simulink model "Lab8_model_12a"  (R2012a)
settings: Solver=ode45  StartTime=0.0  StopTime=20  RelTol=1e-3
values from neighbouring files (symbols this model uses):
  A = [0 4 2;0 0 2;6 2 3]    [Lab8.m]
  B = [3;0;0]    [Lab8.m]
  C = [4 1 2]    [Lab8.m]
  D = 0    [Lab8.m]
  K = 0.02    [Controle_Lab4.m]    (also in Lab8.m = place(A,B,[-10 -12 -2]); Tarefa1.m)
  K1 = 9    [Lab8.m]
  K2 = 11    [Lab8.m]
  K3 = 14.5    [Lab8.m]
settings Model: Creator=11104980  LastModifiedBy=Jessica
settings DataIOCC: LimitDataPoints=on  SaveFormat=Array  ReturnWorkspaceOutputs=off
settings OptimizationCC: ExpressionDepthLimit=2147483647  LifeSpan=inf  SimCompilerOptimization=Off
settings DebuggingCC: UnderspecifiedInitializationDetection=Classic  MergeDetectMultiDrivingBlocksExec=none  FcnCallInpInsideContextMsg=Enable All  StateNameClashWarn=warning  SFUnexpectedBacktrackingDiag=warning  SFNoUnconditionalDefaultTransitionDiag=warning
settings HardwareCC: ProdBitPerPointer=32  ProdLargestAtomicFloat=None  ProdIntDivRoundTo=Undefined  ProdEndianess=Unspecified  ProdWordSize=32  ProdHWDeviceType=32-bit Generic
settings ModelReferenceCC: PropagateSignalLabelsOutOfModel=off
settings SFSimCC: SimUseLocalCustomCode=off
settings RTWCC: RTWUseLocalCustomCode=off  RTWCompilerOptimization=Off
settings GRTTargetCC: CodeReplacementLibrary=C89/C90 (ANSI)  GeneratePreprocessorConditionals=Disable all  CPPClassGenCompliant=off

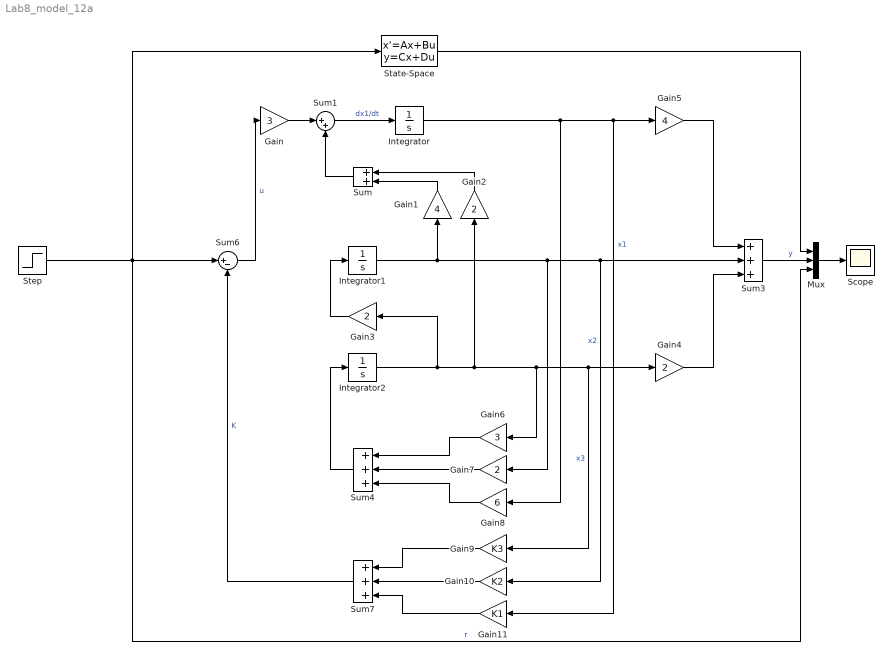
== system Lab8_model_12a ==
  Gain : Gain  Gain=3
  Gain1 : Gain  Gain=4
  Gain10 : Gain  Gain=K2
  Gain11 : Gain  Gain=K1
  Gain{2..4,7} (4 alike) : Gain  Gain=2
  Gain5 : Gain  Gain=4
  Gain6 : Gain  Gain=3
  Gain8 : Gain  Gain=6
  Gain9 : Gain  Gain=K3
  Integrator : Integrator
  Integrator1 : Integrator
  Integrator2 : Integrator
  Mux : Mux  Inputs=3
  Scope : Scope
      settings: SaveName=y
  State-Space : StateSpace  A=(A-B*K)  B=B  C=C  D=D  X0=0
  Step : Step  SampleTime=0
  Sum : Sum
  Sum1 : Sum  Inputs=|++
  Sum3 : Sum  Inputs=+++
  Sum4 : Sum  Inputs=+++
  Sum6 : Sum  Inputs=|+-
  Sum7 : Sum  Inputs=+++
  wires:
  Sum/1 -> Sum1/2
  Gain/1 -> Sum1/1
  Sum1/1 -> Integrator/1  "dx1/dt"
  Gain1/1 -> Sum/2
  Gain2/1 -> Sum/1
  Integrator1/1 -> Sum3/2, Gain10/1, Gain7/1, Gain1/1  "x2"
  Integrator2/1 -> Gain6/1, Gain9/1, Gain4/1, Gain2/1, Gain3/1  "x3"
  Integrator/1 -> Gain5/1, Gain11/1, Gain8/1  "x1"
  Gain5/1 -> Sum3/1
  Gain4/1 -> Sum3/3
  Gain7/1 -> Sum4/2
  Gain6/1 -> Sum4/1
  Gain8/1 -> Sum4/3
  Step/1 -> Sum6/1, State-Space/1, Mux/3  "r"
  Sum6/1 -> Gain/1  "u"
  Gain10/1 -> Sum7/2
  Gain9/1 -> Sum7/1
  Gain11/1 -> Sum7/3
  Sum7/1 -> Sum6/2  "K"
  Mux/1 -> Scope/1
  State-Space/1 -> Mux/1
  Sum3/1 -> Mux/2  "y"
  Gain3/1 -> Integrator1/1
  Sum4/1 -> Integrator2/1
